simulink model "MainModel"  (R2020b)
settings: Solver=VariableStepAuto  StartTime=0.0  StopTime=inf  RelTol=1e-3
settings Model: Creator=tomonori  LastModifiedBy=tomonori

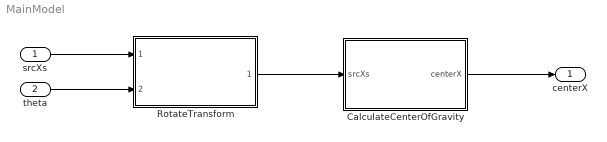
== system MainModel ==
  srcXs : Inport
  theta : Inport  Port=2
  CalculateCenterOfGravity : Subsystem
  RotateTransform : Subsystem  ReferencedSubsystem=RotateTransform
  centerX : Outport
  wires:
  srcXs/1 -> RotateTransform/1
  theta/1 -> RotateTransform/2
  RotateTransform/1 -> CalculateCenterOfGravity/1(srcXs)
  CalculateCenterOfGravity/1(centerX) -> centerX/1

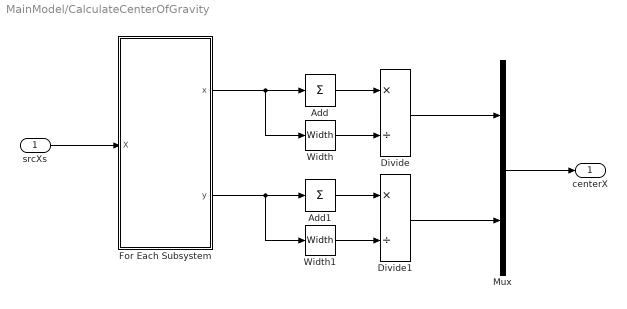
== system MainModel/CalculateCenterOfGravity ==
  srcXs : Inport
  Add : Sum  Inputs=+
  Add1 : Sum  Inputs=+
  Divide : Product  Inputs=*/
  Divide1 : Product  Inputs=*/
  For Each Subsystem : Subsystem  TreatAsAtomicUnit=on
  Mux : Mux  Inputs=2
  Width : Width
  Width1 : Width
  centerX : Outport
  wires:
  srcXs/1 -> For Each Subsystem/1(X)
  For Each Subsystem/1(x) -> Width/1, Add/1
  Width/1 -> Divide/2
  Add/1 -> Divide/1
  Add1/1 -> Divide1/1
  Width1/1 -> Divide1/2
  For Each Subsystem/2(y) -> Width1/1, Add1/1
  Divide1/1 -> Mux/2
  Divide/1 -> Mux/1
  Mux/1 -> centerX/1

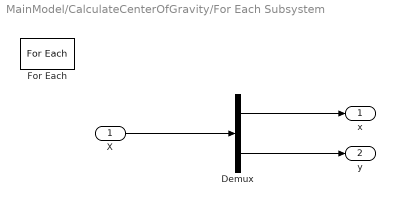
== system MainModel/CalculateCenterOfGravity/For Each Subsystem ==
  X : Inport  Partition=on  PartitionDimension=1  PartitionWidth=1  PartitionOffset=0
  Demux : Demux  Outputs=2
  For Each : ForEach  DisableCoverage=on
  x : Outport  ConcatenationDimension=1
  y : Outport  Port=2  ConcatenationDimension=1
  wires:
  X/1 -> Demux/1
  Demux/1 -> x/1
  Demux/2 -> y/1
